simulink model "DEA_strip_t7"  (R2018a)
settings: Solver=ode23t  StartTime=0.0  StopTime=param_simtime  EnableMultiTasking=on
InitFcn:
  | Parameter;
values from neighbouring files (symbols this model uses):
  param_f = 0.001    [plot_task7.m]    (also in plot_task7_chirp.m)
  param_g = 9.81    [plot_task7.m]    (also in plot_task7_chirp.m)
  param_k1 = -5000    [plot_task7.m]    (also in plot_task7_chirp.m = 10800)
  param_m1 = 0.25    [plot_task7.m]    (also in plot_task7_chirp.m)
  param_N = 8    [plot_task7.m]    (also in plot_task7_chirp.m)
  param_v = 2500    [plot_task7.m]    (also in plot_task7_chirp.m = 0)
  param_ys0 = 0.009    [plot_task7.m]    (also in plot_task7_chirp.m = 0.02)
undefined symbols (not defined in the file or in its folder): params
settings Model: Creator=Johannes  LastModifiedBy=Tim
settings DataIOCC: LimitDataPoints=on  SaveFormat=Array  SignalLoggingSaveFormat=ModelDataLogs
settings OptimizationCC: LifeSpan=inf
settings DebuggingCC: UnderspecifiedInitializationDetection=Classic  MergeDetectMultiDrivingBlocksExec=none  SolverPrmCheckMsg=warning  MultiTaskDSMMsg=warning  MultiTaskCondExecSysMsg=none  SFUnexpectedBacktrackingDiag=warning  SFNoUnconditionalDefaultTransitionDiag=warning  SFExecutionAtInitializationDiag=none
settings HardwareCC: ProdBitPerPointer=32  ProdBitPerSizeT=32  ProdBitPerPtrDiffT=32  ProdLargestAtomicFloat=None  ProdIntDivRoundTo=Undefined  ProdEndianess=Unspecified  ProdWordSize=32  ProdHWDeviceType=32-bit Generic
settings ModelReferenceCC: PropagateSignalLabelsOutOfModel=off
settings CodeAppCC: StateflowObjectComments=on
settings GRTTargetCC: TargetLangStandard=C89/C90 (ANSI)  GeneratePreprocessorConditionals=Disable all
settings ConfigComp: CovMetricSettings=dw  CovHtmlReporting=on  CovSaveCumulativeToWorkspaceVar=on  CovSaveSingleToWorkspaceVar=on  CovExternalEMLEnable=off

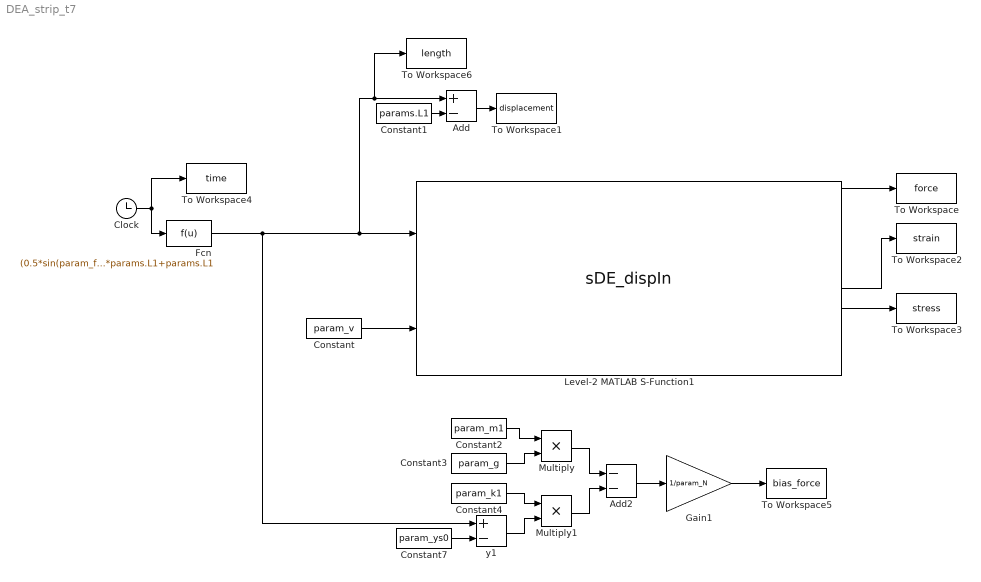
== system DEA_strip_t7 ==
  Add : Sum  Inputs=+-
  Add2 : Sum  Inputs=--
  Clock : Clock
  Constant : Constant  Value=param_v
  Constant1 : Constant  Value=params.L1
  Constant2 : Constant  Value=param_m1
  Constant3 : Constant  Value=param_g
  Constant4 : Constant  Value=param_k1
  Constant7 : Constant  Value=param_ys0
  Fcn : Fcn  Expr=(0.5*sin(param_f*u - pi/2)+0.5)*params.L1+params.L1
  Gain1 : Gain  Gain=1/param_N
  Level-2 MATLAB S-Function1 : M-S-Function  FunctionName=sDE_dispIn  Parameters=params, initConds
      mask Display:
      | color('black');
      | patch(4*[-1 1 1 -1],1.75*[-1 -1 1 1],[1 1 1]);
      | patch(2*[-1 1 1 -1],1.2*[-1 -1 1 1],[0 0 0]);
      | patch(1.95*[-1 1 1 -1],0.8*[-1 -1 1 1],[1 1 1]);
      | disp('DE Actuator');
      | 
      | color('blue');
      | port_label('input', 1, 'l_1 [m]','texmode','on');
      | port_label('input', 2, 'v [V]','texmode','on');
      | 
      | color('red');
      | port_label('output', 1, 'F_1 [N]','texmode','on');
      | port_label('output', 2, 'x_{v1} [-]','texmode','on');
      | port_label('output', 3, 'x_{v2} [-]','texmode','on');
      | port_label('output', 4, '\epsilon_2 [-]','texmode','on');
      | port_label('output', 5, 'q [C]','texmode','on');
      | port_label('output', 6, '\epsilon_1 [-]','texmode','on');
      | port_label('output', 7, '\sigma_1 [Pa]','texmode','on');
      | port_label('output', 8, 'i [A]','texmode','on');
      | port_label('output', 9, 'v_{DE} [V]','texmode','on');
      | port_label('output', 10, 'C [F]','texmode','on');
  Multiply : Product
  Multiply1 : Product
  To Workspace : ToWorkspace  VariableName=force  SampleTime=-1
  To Workspace1 : ToWorkspace  VariableName=displacement  SampleTime=-1
  To Workspace2 : ToWorkspace  VariableName=strain  SampleTime=-1
  To Workspace3 : ToWorkspace  VariableName=stress  SampleTime=-1
  To Workspace4 : ToWorkspace  VariableName=time  SampleTime=-1
  To Workspace5 : ToWorkspace  VariableName=bias_force  SampleTime=-1
  To Workspace6 : ToWorkspace  VariableName=length  SampleTime=-1
  "y1 " : Sum  Inputs=+-
  wires:
  Clock/1 -> Fcn/1, To Workspace4/1
  Fcn/1 -> "y1 "/1, To Workspace6/1, Add/1, Level-2 MATLAB S-Function1/1
  Constant/1 -> Level-2 MATLAB S-Function1/2
  Level-2 MATLAB S-Function1/6 -> To Workspace2/1
  Add/1 -> To Workspace1/1
  Constant1/1 -> Add/2
  Level-2 MATLAB S-Function1/1 -> To Workspace/1
  Constant2/1 -> Multiply/1
  Constant3/1 -> Multiply/2
  Multiply/1 -> Add2/1
  Multiply1/1 -> Add2/2
  Constant4/1 -> Multiply1/1
  "y1 "/1 -> Multiply1/2
  Constant7/1 -> "y1 "/2
  Add2/1 -> Gain1/1
  Gain1/1 -> To Workspace5/1
  Level-2 MATLAB S-Function1/7 -> To Workspace3/1
